simulink model "bicycle_estimator"  (R2017b)
settings: Solver=FixedStepDiscrete  StartTime=0.0  StopTime=T  FixedStep=0.01  RelTol=1e-3
values from neighbouring files (symbols this model uses):
  Cf = 100000    [Init_for_washout_filter.m]
  Cr = 100000    [Init_for_washout_filter.m]
  L = lf+lr    (= 2.55)    [Init_for_washout_filter.m]
  lf = 0.41*2.55    (= 1.0455)    [Init_for_washout_filter.m]
  lr = 2.55-lf    (= 1.5045)    [Init_for_washout_filter.m]
  mass = 1435-80    (= 1355)    [Init_for_washout_filter.m]
settings Model: Creator=gandh  LastModifiedBy=gandh

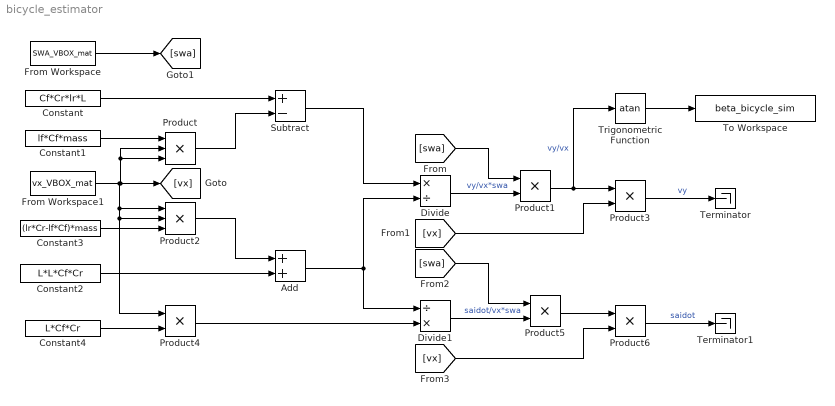
== system bicycle_estimator ==
  Add : Sum
  Constant : Constant  Value=Cf*Cr*lr*L
  Constant1 : Constant  Value=lf*Cf*mass
  Constant2 : Constant  Value=L*L*Cf*Cr
  Constant3 : Constant  Value=(lr*Cr-lf*Cf)*mass
  Constant4 : Constant  Value=L*Cf*Cr
  Divide : Product  Inputs=*/
  Divide1 : Product  Inputs=/*
  From Workspace : FromWorkspace  VariableName=SWA_VBOX_mat  SampleTime=0
  From Workspace1 : FromWorkspace  VariableName=vx_VBOX_mat  SampleTime=0
  Product : Product  Inputs=3
  Product{1,3..6} (5 alike) : Product
  Product2 : Product  Inputs=3
  Subtract : Sum  Inputs=+-
  Terminator : Terminator
  Terminator1 : Terminator
  To Workspace : ToWorkspace  VariableName=beta_bicycle_sim  SaveFormat=Timeseries  SampleTime=-1
  Trigonometric Function : Trigonometry  Operator=atan
  wires:
  From Workspace1/1 -> Product2/2, Product4/1, Product2/1, [vx], Product/3, Product/2
  Constant1/1 -> Product/1
  Constant/1 -> Subtract/1
  Product/1 -> Subtract/2
  Constant3/1 -> Product2/3
  Product2/1 -> Add/1
  Constant2/1 -> Add/2
  Subtract/1 -> Divide/1
  Add/1 -> Divide1/1, Divide/2
  Divide/1 -> Product1/2  "vy/vx*swa"
  [swa] -> Product1/1
  Product1/1 -> Trigonometric Function/1, Product3/1  "vy/vx"
  From Workspace/1 -> [swa]
  [vx] -> Product3/2
  Product3/1 -> Terminator/1  "vy"
  Trigonometric Function/1 -> To Workspace/1
  Constant4/1 -> Product4/2
  Product4/1 -> Divide1/2
  Divide1/1 -> Product5/2  "saidot/vx*swa"
  [swa] -> Product5/1
  [vx] -> Product6/2
  Product5/1 -> Product6/1
  Product6/1 -> Terminator1/1  "saidot"
